simulink model "Full_Model_5"  (R2018b)
settings: Solver=VariableStepAuto  StartTime=0.0  StopTime=.5  RelTol=1e-3
InitFcn:
  | Robot_Body_Constants
values from neighbouring files (symbols this model uses):
  robot_radius = 0.0789    [Robot_Body_Constants.m]
  wheel_angles = [pi * 0.25 pi * 0.75 pi * 1.25 pi * 1.75]    [Robot_Body_Constants.m]
libraries: powerlib x56, peBldcCurrentController x4, simulink x1, dspinverses x1
(part 2 of 2)

== matlab function Full_Model_5/Inverse Dynamics ==
  data: v input; u output; a input; phi input; Jl input; Jm input; cl input; cm input; G input; gear_ratio input; M input; wheel_radius input; gRb input
function u = inverse_dynamics(v, a, phi, Jl, Jm, cl, cm, G, gear_ratio, M, wheel_radius, gRb)
    phidot = v(3, 1); %Double check this
    I4 = eye(4);
    GTinv = pinv(G');
    Ginv = pinv(G);
    %gRb = rotation_matrix(phi);
    w_l = G' * gRb' * v / wheel_radius;
    
    Rdot = -phidot * [-sin(phi), -cos(phi), 0; cos(phi), sin(phi), 0; 0, 0, 0];
    RTRdot = phidot * [0 1 0; -1 0 0; 0 0 0];
    
    Z = (((Jm + Jl) / gear_ratio^2) * I4) + (wheel_radius^2/gear_ratio^2) * (Ginv * M) * GTinv;
    v = ((cm + cl / gear_ratio^2) * I4) + (wheel_radius^2/gear_ratio^2) * (Ginv * RTRdot) * GTinv;
    
    wldot = (G' * gRb' / wheel_radius) * (a - Rdot * GTinv * wheel_radius * w_l);
    A = -pinv(Z) * v;
    u = Z * gear_ratio * (wldot - A * w_l);
end

== matlab function Full_Model_5/Rotation Matrix ==
  data: phi input; rot output
function rot = rotation_matrix(phi)
    rot = [cos(phi) -sin(phi) 0; sin(phi) cos(phi) 0; 0 0 1];
end
